simulink subsystem "iteration"  (R2022a)
settings: Solver=VariableStepAuto  StartTime=0.0  StopTime=10.0  RelTol=1e-3
settings Model: Creator=lsfan  LastModifiedBy=lsfan

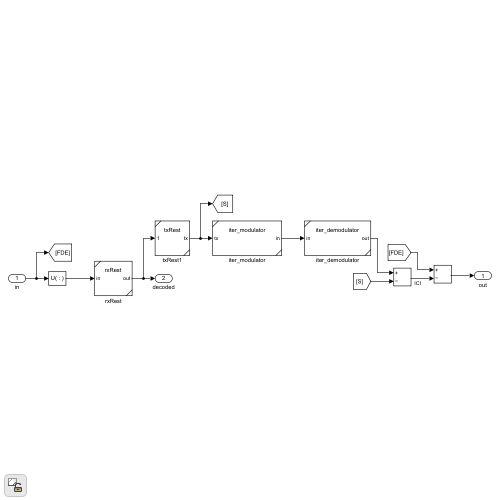
[thumbnail: Simulink's stored preview of the top-level diagram]
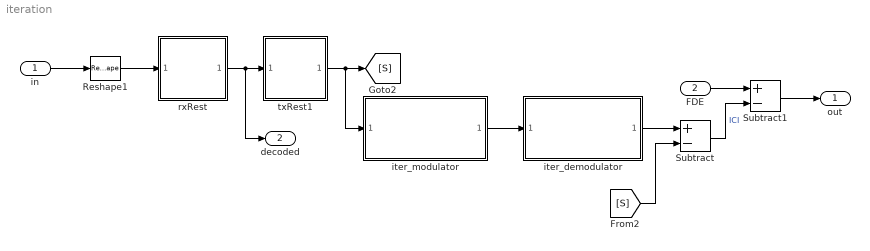
== system iteration ==
  in : Inport
  FDE : Inport  Port=2
  Reshape1 : Reshape
  Subtract : Sum  Inputs=+-
  Subtract1 : Sum  Inputs=+-
  iter_demodulator : Subsystem  ReferencedSubsystem=iter_demodulator
  iter_modulator : Subsystem  ReferencedSubsystem=iter_modulator
  rxRest : Subsystem  ReferencedSubsystem=rxRest
  txRest1 : Subsystem  ReferencedSubsystem=txRest
  out : Outport
  decoded : Outport  Port=2
  wires:
  iter_demodulator/1 -> Subtract/1
  in/1 -> Reshape1/1
  FDE/1 -> Subtract1/1
  iter_modulator/1 -> iter_demodulator/1
  Subtract1/1 -> out/1
  Reshape1/1 -> rxRest/1
  Subtract/1 -> Subtract1/2  "ICI"
  [S] -> Subtract/2
  rxRest/1 -> decoded/1, txRest1/1
  txRest1/1 -> iter_modulator/1, [S]
